simulink model "TrajectoryTracking_2015b_00"  (R2017a)
settings: Solver=ode45  StartTime=0.0  StopTime=200  RelTol=1e-3
values from neighbouring files (symbols this model uses):
  tau_d_1 = C_RB1+C_A1+D1+G1    [DesiredInputOptimalConfiguration.m]
  tau_d_2 = C_RB2+C_A2+D2+G2    [DesiredInputOptimalConfiguration.m]
  tau_d_3 = C_RB3+C_A3+D3+G3    [DesiredInputOptimalConfiguration.m]
  tau_d_4 = C_RB4+C_A4+D4+G4    [DesiredInputOptimalConfiguration.m]
  tau_d_5 = C_RB5+C_A5+D5+G5    [DesiredInputOptimalConfiguration.m]
  tau_d_6 = C_RB6+C_A6+D6+G6    [DesiredInputOptimalConfiguration.m]
  tau_d_7 = C_RB7+C_A7+D7+G7    [DesiredInputOptimalConfiguration.m]
undefined symbols (not defined in the file or in its folder): angular_velocity_pitch_1, angular_velocity_pitch_2, angular_velocity_pitch_3, angular_velocity_pitch_4, angular_velocity_pitch_5, angular_velocity_pitch_6, angular_velocity_roll_1, angular_velocity_roll_2, angular_velocity_roll_3, angular_velocity_roll_4, angular_velocity_roll_5, angular_velocity_roll_6, angular_velocity_roll_7, angular_velocity_yaw_1, angular_velocity_yaw_2, angular_velocity_yaw_3, angular_velocity_yaw_4, angular_velocity_yaw_5, angular_velocity_yaw_6, angular_velocity_yaw_7, B_input, d_H, K1, K2, K3, K4, K5, K6, K7, linear_velocity_x_1, linear_velocity_x_2, linear_velocity_x_3, linear_velocity_x_4, linear_velocity_x_5, linear_velocity_x_6, linear_velocity_x_7, linear_velocity_y_1, linear_velocity_y_2, linear_velocity_y_3, linear_velocity_y_4, linear_velocity_y_5, linear_velocity_y_6, linear_velocity_y_7, linear_velocity_z_1, linear_velocity_z_2, linear_velocity_z_3, linear_velocity_z_4, linear_velocity_z_5, linear_velocity_z_6, linear_velocity_z_7, pitch_angle_1, pitch_angle_2, pitch_angle_3, pitch_angle_4, pitch_angle_5, pitch_angle_6, pitch_angle_7, roll_angle_1, roll_angle_2, roll_angle_3 ... (+54)
undefined symbols (not defined in the file): a_F2, a_F3, a_F4, b_F2, b_F3, b_F4, b_T1_optimized, b_T2_optimized, b_T3_optimized, b_T4_optimized, b_T5_optimized, b_T6_optimized, d_T1_optimized, d_T2_optimized, d_T3_optimized, d_T4_optimized, d_T5_optimized, d_T6_optimized, gamma_F1_optimized, gamma_F2_optimized, gamma_F3_optimized, gamma_F4_optimized, r_T1_optimized, r_T2_optimized, r_T3_optimized, r_T4_optimized, r_T5_optimized, r_T6_optimized, x_F1_optimized, x_F2_optimized, x_F3_optimized, x_F4_optimized
libraries: sharedtransform x1, shared6dofsys x1
(part 2 of 3)

== system TrajectoryTracking_2015b_00/Nonlinear Transformation/Velocity Error /sway_error ==
  sway : Inport
  SwitchSchedule : Inport  Port=2
  Scope3 : Scope  NumInputPorts=2
  Sum5 : Sum  Inputs=|+-
  sway_d : Subsystem
  sway_err : Outport
  wires:
  sway/1 -> Sum5/1
  Sum5/1 -> Scope3/1, sway_err/1
  SwitchSchedule/1 -> sway_d/1(SwitchSchedule)
  sway_d/1(sway_d) -> Scope3/2, Sum5/2

== system TrajectoryTracking_2015b_00/Nonlinear Transformation/Velocity Error /yaw_error ==
  pitch : Inport
  SwitchSchedule : Inport  Port=2
  Scope1 : Scope  NumInputPorts=2
  Scope3 : Scope  NumInputPorts=2
  Sum5 : Sum  Inputs=|+-
  yaw_d : Subsystem
  pitch_err : Outport
  wires:
  pitch/1 -> Scope1/1, Scope3/1, Sum5/1
  Sum5/1 -> pitch_err/1
  yaw_d/1(yaw_d) -> Sum5/2, Scope1/2, Scope3/2
  SwitchSchedule/1 -> yaw_d/1(SwitchSchedule)

== system TrajectoryTracking_2015b_00/Underwater Robot System/Underwater Robot System/DragCalculation ==
  nu : Inport
  Abs : Abs
  Constant : Constant  Value=veh.D
  Product : Product  Multiplication=Matrix(*)
  Product1 : Product
  HullDrag : Outport
  wires:
  Product/1 -> HullDrag/1
  Product1/1 -> Product/2
  Abs/1 -> Product1/1
  Constant/1 -> Product/1
  nu/1 -> Abs/1, Product1/2  "nu"

== system TrajectoryTracking_2015b_00/Underwater Robot System/Underwater Robot System/Dynamic2Kinematic(angular velocity) ==
  "p q r " : Inport
  Initial Integration Phi : Subsystem
  Initial Integration Value Generation Psi : Subsystem
  Initial Integration Value Generation Theta : Subsystem
  Mux1 : Mux  Inputs=3
  Rotation Angles to Direction Cosine Matrix : sharedtransform/Rotation Angles to Direction Cosine Matrix  rotationOrder=ZYX
      settings: SourceProductBaseCode=AE
  Selector : Selector  InputPortWidth=3  IndexOptions=Index vector (dialog)  Indices=[3 2 1]  OutputSizes=1
  phi theta psi : Integrator  InitialConditionSource=external
  phidot thetadot psidot : shared6dofsys/DCM & Euler Angles (Euler)/phidot thetadot psidot
  DCM : Outport
  Euler : Outport  Port=2
  Euler_dot : Outport  Port=3
  wires:
  Selector/1 -> Rotation Angles to Direction Cosine Matrix/1
  "p q r "/1 -> phidot thetadot psidot/1
  phi theta psi/1 -> phidot thetadot psidot/2, Selector/1, Euler/1
  phidot thetadot psidot/1 -> Euler_dot/1, phi theta psi/1
  Rotation Angles to Direction Cosine Matrix/1 -> DCM/1
  Initial Integration Value Generation Psi/1(Initial Orientation Integration Value) -> Mux1/3
  Initial Integration Value Generation Theta/1(Initial Theta Integration Value) -> Mux1/2
  Mux1/1 -> phi theta psi/2
  Initial Integration Phi/1(Initial Phi Integration Value) -> Mux1/1

== system TrajectoryTracking_2015b_00/Underwater Robot System/Underwater Robot System/Initial Integration Value Generation Generalised Location ==
  Constant : Constant  Value=0
  Mux : Mux  Inputs=3
  Initial Location Integration Value : Outport
  wires:
  Constant/1 -> Mux/1, Mux/3, Mux/2
  Mux/1 -> Initial Location Integration Value/1

== system TrajectoryTracking_2015b_00/Underwater Robot System/Underwater Robot System/Underwater Robot Dynamics  ==
  tau_b : Inport
  6DOF Coriolis forces : Subsystem
  M_A : Constant  Value=veh.Ma
  M_RB : Constant  Value=veh.Mrb
  Product : Product  Inputs=/*  Multiplication=Matrix(*)  SaturateOnIntegerOverflow=on  OutDataTypeStr=Inherit: Same as first input
  Scope : Scope
  Selector1 : Selector  InputPortWidth=6  IndexOptions=Index vector (dialog)  Indices=[1 2 3]  OutputSizes=1
  Selector2 : Selector  InputPortWidth=6  IndexOptions=Index vector (dialog)  Indices=[4 5 6]  OutputSizes=1
  Sum : Sum  Inputs=|+-
  Sum2 : Sum  SaturateOnIntegerOverflow=on
  Velocity Integrator : Integrator
  v : Outport
  w_ib : Outport  Port=2
  wires:
  M_RB/1 -> Sum2/1
  M_A/1 -> Sum2/2
  Sum2/1 -> Product/1, 6DOF Coriolis forces/1(M)  "M"
  Selector2/1 -> w_ib/1  "w_nb"
  Product/1 -> Velocity Integrator/1  "(d/dt)nu"
  6DOF Coriolis forces/1(C(nu)nu) -> Sum/2, Scope/1
  Sum/1 -> Product/2
  Selector1/1 -> v/1  "v"
  Velocity Integrator/1 -> 6DOF Coriolis forces/2(nu), Selector2/1, Selector1/1  "nu"
  tau_b/1 -> Sum/1

== system TrajectoryTracking_2015b_00/Underwater Robot System/Underwater Robot System/transform to inertial world frame {i} ==
  v : Inport
  linear velocity transformation matrix : Inport  Port=2
  Product : Product  Multiplication=Matrix(*)  SaturateOnIntegerOverflow=on  InputSameDT=on  OutDataTypeStr=Inherit: Same as first input
  Reshape1 : Reshape  OutputDimensionality=Column vector (2-D)
  Reshape2 : Reshape
  Ve : Outport
  wires:
  Product/1 -> Reshape2/1
  Reshape1/1 -> Product/2
  v/1 -> Reshape1/1
  Reshape2/1 -> Ve/1
  linear velocity transformation matrix/1 -> Product/1

== system TrajectoryTracking_2015b_00/Actuator1/Simplified Fin Model 1/Drag Forces and Moments/3x3 cross product ==
  a : Inport
  b : Inport  Port=2
  Product : Product  SaturateOnIntegerOverflow=on  InputSameDT=on  OutDataTypeStr=Inherit: Same as first input
  Product1 : Product  SaturateOnIntegerOverflow=on  InputSameDT=on  OutDataTypeStr=Inherit: Same as first input
  Selector : Selector  InputPortWidth=3  IndexOptions=Index vector (dialog)  Indices=[2 3 1]  OutputSizes=1
  Selector1 : Selector  InputPortWidth=3  IndexOptions=Index vector (dialog)  Indices=[3 1 2]  OutputSizes=1
  Selector2 : Selector  InputPortWidth=3  IndexOptions=Index vector (dialog)  Indices=[2 3 1]  OutputSizes=1
  Selector3 : Selector  InputPortWidth=3  IndexOptions=Index vector (dialog)  Indices=[3 1 2]  OutputSizes=1
  Sum : Sum  Inputs=+|-  SaturateOnIntegerOverflow=on  InputSameDT=on  OutDataTypeStr=Inherit: Same as first input
  c : Outport  InitialOutput=0
  wires:
  Selector3/1 -> Product1/1
  Selector2/1 -> Product1/2
  Product1/1 -> Sum/2
  Selector1/1 -> Product/2
  Product/1 -> Sum/1
  a/1 -> Selector3/1, Selector/1
  Selector/1 -> Product/1
  b/1 -> Selector2/1, Selector1/1
  Sum/1 -> c/1

== system TrajectoryTracking_2015b_00/Actuator1/Simplified Fin Model 1/Drag Forces and Moments/Drag Force  ==
  AoA : Inport
  u : Inport  Port=2
  Constant : Constant  Value=0
  Gain1 : Gain  Gain=C_D*a_F*b_F
  Mux : Mux  Inputs=3
  Product : Product  Inputs=3
  q(V_ind) : Subsystem
  Drag Force : Outport
  wires:
  Mux/1 -> Drag Force/1
  Gain1/1 -> Product/1
  q(V_ind)/1(q(V_ind)) -> Gain1/1
  Product/1 -> Mux/1
  u/1 -> q(V_ind)/1(u)
  Constant/1 -> Mux/2, Mux/3
  AoA/1 -> Product/3, Product/2

== system TrajectoryTracking_2015b_00/Actuator1/Simplified Fin Model 1/Drag Forces and Moments/Geometric Center of fin ==
  Constant : Constant  Value=gama_F
  Gain : Gain  Gain=0.5*(d_H+a_F)
  Gain1 : Gain  Gain=0.5*(d_H+a_F)
  Mux : Mux  Inputs=3
  Trigonometric Function : Trigonometry  Operator=cos
  Trigonometric Function1 : Trigonometry
  x_F : Constant  Value=x_F
  r_F : Outport
  wires:
  x_F/1 -> Mux/1
  Constant/1 -> Trigonometric Function/1, Trigonometric Function1/1
  Mux/1 -> r_F/1
  Gain/1 -> Mux/2
  Trigonometric Function1/1 -> Gain/1
  Trigonometric Function/1 -> Gain1/1
  Gain1/1 -> Mux/3

== system TrajectoryTracking_2015b_00/Actuator1/Simplified Fin Model 1/Lift Forces and Moments/3x3 cross product ==
  a : Inport
  b : Inport  Port=2
  Product : Product  SaturateOnIntegerOverflow=on  InputSameDT=on  OutDataTypeStr=Inherit: Same as first input
  Product1 : Product  SaturateOnIntegerOverflow=on  InputSameDT=on  OutDataTypeStr=Inherit: Same as first input
  Selector : Selector  InputPortWidth=3  IndexOptions=Index vector (dialog)  Indices=[2 3 1]  OutputSizes=1
  Selector1 : Selector  InputPortWidth=3  IndexOptions=Index vector (dialog)  Indices=[3 1 2]  OutputSizes=1
  Selector2 : Selector  InputPortWidth=3  IndexOptions=Index vector (dialog)  Indices=[2 3 1]  OutputSizes=1
  Selector3 : Selector  InputPortWidth=3  IndexOptions=Index vector (dialog)  Indices=[3 1 2]  OutputSizes=1
  Sum : Sum  Inputs=+|-  SaturateOnIntegerOverflow=on  InputSameDT=on  OutDataTypeStr=Inherit: Same as first input
  c : Outport  InitialOutput=0
  wires:
  Selector3/1 -> Product1/1
  Selector2/1 -> Product1/2
  Product1/1 -> Sum/2
  Selector1/1 -> Product/2
  Product/1 -> Sum/1
  a/1 -> Selector3/1, Selector/1
  Selector/1 -> Product/1
  b/1 -> Selector2/1, Selector1/1
  Sum/1 -> c/1

== system TrajectoryTracking_2015b_00/Actuator1/Simplified Fin Model 1/Lift Forces and Moments/Geometric Center of fin ==
  Constant : Constant  Value=gama_F
  Gain : Gain  Gain=0.5*(d_H+a_F)
  Gain1 : Gain  Gain=0.5*(d_H+a_F)
  Mux : Mux  Inputs=3
  Trigonometric Function : Trigonometry  Operator=cos
  Trigonometric Function1 : Trigonometry
  x_F : Constant  Value=x_F
  r_F : Outport
  wires:
  x_F/1 -> Mux/1
  Constant/1 -> Trigonometric Function/1, Trigonometric Function1/1
  Mux/1 -> r_F/1
  Gain/1 -> Mux/2
  Trigonometric Function1/1 -> Gain/1
  Trigonometric Function/1 -> Gain1/1
  Gain1/1 -> Mux/3

== system TrajectoryTracking_2015b_00/Actuator1/Simplified Fin Model 1/Lift Forces and Moments/Lift Force  ==
  u : Inport
  AoA : Inport  Port=2
  Constant : Constant  Value=0
  Constant1 : Constant  Value=gama_F
  Gain1 : Gain  Gain=C_L*a_F*b_F
  Gain2 : Gain  Gain=-C_L*a_F*b_F
  Mux : Mux  Inputs=3
  Product : Product  Inputs=3
  Product1 : Product  Inputs=3
  Trigonometric Function : Trigonometry  Operator=cos
  Trigonometric Function1 : Trigonometry
  q(V_ind) : Subsystem
  Lift Force : Outport
  wires:
  u/1 -> q(V_ind)/1(u)
  q(V_ind)/1(q(V_ind)) -> Gain2/1, Gain1/1
  Gain1/1 -> Product/1
  Trigonometric Function/1 -> Product/2
  Mux/1 -> Lift Force/1
  Gain2/1 -> Product1/1
  Trigonometric Function1/1 -> Product1/2
  Constant/1 -> Mux/1
  Product/1 -> Mux/2
  Product1/1 -> Mux/3
  AoA/1 -> Product/3, Product1/3
  Constant1/1 -> Trigonometric Function1/1, Trigonometric Function/1

== system TrajectoryTracking_2015b_00/Actuator1/Simplified Fin Model 2/Drag Forces and Moments/3x3 cross product ==
  a : Inport
  b : Inport  Port=2
  Product : Product  SaturateOnIntegerOverflow=on  InputSameDT=on  OutDataTypeStr=Inherit: Same as first input
  Product1 : Product  SaturateOnIntegerOverflow=on  InputSameDT=on  OutDataTypeStr=Inherit: Same as first input
  Selector : Selector  InputPortWidth=3  IndexOptions=Index vector (dialog)  Indices=[2 3 1]  OutputSizes=1
  Selector1 : Selector  InputPortWidth=3  IndexOptions=Index vector (dialog)  Indices=[3 1 2]  OutputSizes=1
  Selector2 : Selector  InputPortWidth=3  IndexOptions=Index vector (dialog)  Indices=[2 3 1]  OutputSizes=1
  Selector3 : Selector  InputPortWidth=3  IndexOptions=Index vector (dialog)  Indices=[3 1 2]  OutputSizes=1
  Sum : Sum  Inputs=+|-  SaturateOnIntegerOverflow=on  InputSameDT=on  OutDataTypeStr=Inherit: Same as first input
  c : Outport  InitialOutput=0
  wires:
  Selector3/1 -> Product1/1
  Selector2/1 -> Product1/2
  Product1/1 -> Sum/2
  Selector1/1 -> Product/2
  Product/1 -> Sum/1
  a/1 -> Selector3/1, Selector/1
  Selector/1 -> Product/1
  b/1 -> Selector2/1, Selector1/1
  Sum/1 -> c/1

== system TrajectoryTracking_2015b_00/Actuator1/Simplified Fin Model 2/Drag Forces and Moments/Drag Force  ==
  AoA : Inport
  u : Inport  Port=2
  Constant : Constant  Value=0
  Gain1 : Gain  Gain=C_D*a_F*b_F
  Mux : Mux  Inputs=3
  Product : Product  Inputs=3
  q(V_ind) : Subsystem
  Drag Force : Outport
  wires:
  Mux/1 -> Drag Force/1
  Gain1/1 -> Product/1
  q(V_ind)/1(q(V_ind)) -> Gain1/1
  Product/1 -> Mux/1
  u/1 -> q(V_ind)/1(u)
  Constant/1 -> Mux/2, Mux/3
  AoA/1 -> Product/3, Product/2

== system TrajectoryTracking_2015b_00/Actuator1/Simplified Fin Model 2/Drag Forces and Moments/Geometric Center of fin ==
  Constant : Constant  Value=gama_F
  Gain : Gain  Gain=0.5*(d_H+a_F)
  Gain1 : Gain  Gain=0.5*(d_H+a_F)
  Mux : Mux  Inputs=3
  Trigonometric Function : Trigonometry  Operator=cos
  Trigonometric Function1 : Trigonometry
  x_F : Constant  Value=x_F
  r_F : Outport
  wires:
  x_F/1 -> Mux/1
  Constant/1 -> Trigonometric Function/1, Trigonometric Function1/1
  Mux/1 -> r_F/1
  Gain/1 -> Mux/2
  Trigonometric Function1/1 -> Gain/1
  Trigonometric Function/1 -> Gain1/1
  Gain1/1 -> Mux/3

== system TrajectoryTracking_2015b_00/Actuator1/Simplified Fin Model 2/Lift Forces and Moments/3x3 cross product ==
  a : Inport
  b : Inport  Port=2
  Product : Product  SaturateOnIntegerOverflow=on  InputSameDT=on  OutDataTypeStr=Inherit: Same as first input
  Product1 : Product  SaturateOnIntegerOverflow=on  InputSameDT=on  OutDataTypeStr=Inherit: Same as first input
  Selector : Selector  InputPortWidth=3  IndexOptions=Index vector (dialog)  Indices=[2 3 1]  OutputSizes=1
  Selector1 : Selector  InputPortWidth=3  IndexOptions=Index vector (dialog)  Indices=[3 1 2]  OutputSizes=1
  Selector2 : Selector  InputPortWidth=3  IndexOptions=Index vector (dialog)  Indices=[2 3 1]  OutputSizes=1
  Selector3 : Selector  InputPortWidth=3  IndexOptions=Index vector (dialog)  Indices=[3 1 2]  OutputSizes=1
  Sum : Sum  Inputs=+|-  SaturateOnIntegerOverflow=on  InputSameDT=on  OutDataTypeStr=Inherit: Same as first input
  c : Outport  InitialOutput=0
  wires:
  Selector3/1 -> Product1/1
  Selector2/1 -> Product1/2
  Product1/1 -> Sum/2
  Selector1/1 -> Product/2
  Product/1 -> Sum/1
  a/1 -> Selector3/1, Selector/1
  Selector/1 -> Product/1
  b/1 -> Selector2/1, Selector1/1
  Sum/1 -> c/1

== system TrajectoryTracking_2015b_00/Actuator1/Simplified Fin Model 2/Lift Forces and Moments/Geometric Center of fin ==
  Constant : Constant  Value=gama_F
  Gain : Gain  Gain=0.5*(d_H+a_F)
  Gain1 : Gain  Gain=0.5*(d_H+a_F)
  Mux : Mux  Inputs=3
  Trigonometric Function : Trigonometry  Operator=cos
  Trigonometric Function1 : Trigonometry
  x_F : Constant  Value=x_F
  r_F : Outport
  wires:
  x_F/1 -> Mux/1
  Constant/1 -> Trigonometric Function/1, Trigonometric Function1/1
  Mux/1 -> r_F/1
  Gain/1 -> Mux/2
  Trigonometric Function1/1 -> Gain/1
  Trigonometric Function/1 -> Gain1/1
  Gain1/1 -> Mux/3

== system TrajectoryTracking_2015b_00/Actuator1/Simplified Fin Model 2/Lift Forces and Moments/Lift Force  ==
  u : Inport
  AoA : Inport  Port=2
  Constant : Constant  Value=0
  Constant1 : Constant  Value=gama_F
  Gain1 : Gain  Gain=C_L*a_F*b_F
  Gain2 : Gain  Gain=-C_L*a_F*b_F
  Mux : Mux  Inputs=3
  Product : Product  Inputs=3
  Product1 : Product  Inputs=3
  Trigonometric Function : Trigonometry  Operator=cos
  Trigonometric Function1 : Trigonometry
  q(V_ind) : Subsystem
  Lift Force : Outport
  wires:
  u/1 -> q(V_ind)/1(u)
  q(V_ind)/1(q(V_ind)) -> Gain2/1, Gain1/1
  Gain1/1 -> Product/1
  Trigonometric Function/1 -> Product/2
  Mux/1 -> Lift Force/1
  Gain2/1 -> Product1/1
  Trigonometric Function1/1 -> Product1/2
  Constant/1 -> Mux/1
  Product/1 -> Mux/2
  Product1/1 -> Mux/3
  AoA/1 -> Product/3, Product1/3
  Constant1/1 -> Trigonometric Function1/1, Trigonometric Function/1

== system TrajectoryTracking_2015b_00/Actuator1/Simplified Fin Model 3/Drag Forces and Moments/3x3 cross product ==
  a : Inport
  b : Inport  Port=2
  Product : Product  SaturateOnIntegerOverflow=on  InputSameDT=on  OutDataTypeStr=Inherit: Same as first input
  Product1 : Product  SaturateOnIntegerOverflow=on  InputSameDT=on  OutDataTypeStr=Inherit: Same as first input
  Selector : Selector  InputPortWidth=3  IndexOptions=Index vector (dialog)  Indices=[2 3 1]  OutputSizes=1
  Selector1 : Selector  InputPortWidth=3  IndexOptions=Index vector (dialog)  Indices=[3 1 2]  OutputSizes=1
  Selector2 : Selector  InputPortWidth=3  IndexOptions=Index vector (dialog)  Indices=[2 3 1]  OutputSizes=1
  Selector3 : Selector  InputPortWidth=3  IndexOptions=Index vector (dialog)  Indices=[3 1 2]  OutputSizes=1
  Sum : Sum  Inputs=+|-  SaturateOnIntegerOverflow=on  InputSameDT=on  OutDataTypeStr=Inherit: Same as first input
  c : Outport  InitialOutput=0
  wires:
  Selector3/1 -> Product1/1
  Selector2/1 -> Product1/2
  Product1/1 -> Sum/2
  Selector1/1 -> Product/2
  Product/1 -> Sum/1
  a/1 -> Selector3/1, Selector/1
  Selector/1 -> Product/1
  b/1 -> Selector2/1, Selector1/1
  Sum/1 -> c/1

== system TrajectoryTracking_2015b_00/Actuator1/Simplified Fin Model 3/Drag Forces and Moments/Drag Force  ==
  AoA : Inport
  u : Inport  Port=2
  Constant : Constant  Value=0
  Gain1 : Gain  Gain=C_D*a_F*b_F
  Mux : Mux  Inputs=3
  Product : Product  Inputs=3
  q(V_ind) : Subsystem
  Drag Force : Outport
  wires:
  Mux/1 -> Drag Force/1
  Gain1/1 -> Product/1
  q(V_ind)/1(q(V_ind)) -> Gain1/1
  Product/1 -> Mux/1
  u/1 -> q(V_ind)/1(u)
  Constant/1 -> Mux/2, Mux/3
  AoA/1 -> Product/3, Product/2

== system TrajectoryTracking_2015b_00/Actuator1/Simplified Fin Model 3/Drag Forces and Moments/Geometric Center of fin ==
  Constant : Constant  Value=gama_F
  Gain : Gain  Gain=0.5*(d_H+a_F)
  Gain1 : Gain  Gain=0.5*(d_H+a_F)
  Mux : Mux  Inputs=3
  Trigonometric Function : Trigonometry  Operator=cos
  Trigonometric Function1 : Trigonometry
  x_F : Constant  Value=x_F
  r_F : Outport
  wires:
  x_F/1 -> Mux/1
  Constant/1 -> Trigonometric Function/1, Trigonometric Function1/1
  Mux/1 -> r_F/1
  Gain/1 -> Mux/2
  Trigonometric Function1/1 -> Gain/1
  Trigonometric Function/1 -> Gain1/1
  Gain1/1 -> Mux/3

== system TrajectoryTracking_2015b_00/Actuator1/Simplified Fin Model 3/Lift Forces and Moments/3x3 cross product ==
  a : Inport
  b : Inport  Port=2
  Product : Product  SaturateOnIntegerOverflow=on  InputSameDT=on  OutDataTypeStr=Inherit: Same as first input
  Product1 : Product  SaturateOnIntegerOverflow=on  InputSameDT=on  OutDataTypeStr=Inherit: Same as first input
  Selector : Selector  InputPortWidth=3  IndexOptions=Index vector (dialog)  Indices=[2 3 1]  OutputSizes=1
  Selector1 : Selector  InputPortWidth=3  IndexOptions=Index vector (dialog)  Indices=[3 1 2]  OutputSizes=1
  Selector2 : Selector  InputPortWidth=3  IndexOptions=Index vector (dialog)  Indices=[2 3 1]  OutputSizes=1
  Selector3 : Selector  InputPortWidth=3  IndexOptions=Index vector (dialog)  Indices=[3 1 2]  OutputSizes=1
  Sum : Sum  Inputs=+|-  SaturateOnIntegerOverflow=on  InputSameDT=on  OutDataTypeStr=Inherit: Same as first input
  c : Outport  InitialOutput=0
  wires:
  Selector3/1 -> Product1/1
  Selector2/1 -> Product1/2
  Product1/1 -> Sum/2
  Selector1/1 -> Product/2
  Product/1 -> Sum/1
  a/1 -> Selector3/1, Selector/1
  Selector/1 -> Product/1
  b/1 -> Selector2/1, Selector1/1
  Sum/1 -> c/1

== system TrajectoryTracking_2015b_00/Actuator1/Simplified Fin Model 3/Lift Forces and Moments/Geometric Center of fin ==
  Constant : Constant  Value=gama_F
  Gain : Gain  Gain=0.5*(d_H+a_F)
  Gain1 : Gain  Gain=0.5*(d_H+a_F)
  Mux : Mux  Inputs=3
  Trigonometric Function : Trigonometry  Operator=cos
  Trigonometric Function1 : Trigonometry
  x_F : Constant  Value=x_F
  r_F : Outport
  wires:
  x_F/1 -> Mux/1
  Constant/1 -> Trigonometric Function/1, Trigonometric Function1/1
  Mux/1 -> r_F/1
  Gain/1 -> Mux/2
  Trigonometric Function1/1 -> Gain/1
  Trigonometric Function/1 -> Gain1/1
  Gain1/1 -> Mux/3

== system TrajectoryTracking_2015b_00/Actuator1/Simplified Fin Model 3/Lift Forces and Moments/Lift Force  ==
  u : Inport
  AoA : Inport  Port=2
  Constant : Constant  Value=0
  Constant1 : Constant  Value=gama_F
  Gain1 : Gain  Gain=C_L*a_F*b_F
  Gain2 : Gain  Gain=-C_L*a_F*b_F
  Mux : Mux  Inputs=3
  Product : Product  Inputs=3
  Product1 : Product  Inputs=3
  Trigonometric Function : Trigonometry  Operator=cos
  Trigonometric Function1 : Trigonometry
  q(V_ind) : Subsystem
  Lift Force : Outport
  wires:
  u/1 -> q(V_ind)/1(u)
  q(V_ind)/1(q(V_ind)) -> Gain2/1, Gain1/1
  Gain1/1 -> Product/1
  Trigonometric Function/1 -> Product/2
  Mux/1 -> Lift Force/1
  Gain2/1 -> Product1/1
  Trigonometric Function1/1 -> Product1/2
  Constant/1 -> Mux/1
  Product/1 -> Mux/2
  Product1/1 -> Mux/3
  AoA/1 -> Product/3, Product1/3
  Constant1/1 -> Trigonometric Function1/1, Trigonometric Function/1

== system TrajectoryTracking_2015b_00/Actuator1/Simplified Fin Model 4/Drag Forces and Moments/3x3 cross product ==
  a : Inport
  b : Inport  Port=2
  Product : Product  SaturateOnIntegerOverflow=on  InputSameDT=on  OutDataTypeStr=Inherit: Same as first input
  Product1 : Product  SaturateOnIntegerOverflow=on  InputSameDT=on  OutDataTypeStr=Inherit: Same as first input
  Selector : Selector  InputPortWidth=3  IndexOptions=Index vector (dialog)  Indices=[2 3 1]  OutputSizes=1
  Selector1 : Selector  InputPortWidth=3  IndexOptions=Index vector (dialog)  Indices=[3 1 2]  OutputSizes=1
  Selector2 : Selector  InputPortWidth=3  IndexOptions=Index vector (dialog)  Indices=[2 3 1]  OutputSizes=1
  Selector3 : Selector  InputPortWidth=3  IndexOptions=Index vector (dialog)  Indices=[3 1 2]  OutputSizes=1
  Sum : Sum  Inputs=+|-  SaturateOnIntegerOverflow=on  InputSameDT=on  OutDataTypeStr=Inherit: Same as first input
  c : Outport  InitialOutput=0
  wires:
  Selector3/1 -> Product1/1
  Selector2/1 -> Product1/2
  Product1/1 -> Sum/2
  Selector1/1 -> Product/2
  Product/1 -> Sum/1
  a/1 -> Selector3/1, Selector/1
  Selector/1 -> Product/1
  b/1 -> Selector2/1, Selector1/1
  Sum/1 -> c/1

== system TrajectoryTracking_2015b_00/Actuator1/Simplified Fin Model 4/Drag Forces and Moments/Drag Force  ==
  AoA : Inport
  u : Inport  Port=2
  Constant : Constant  Value=0
  Gain1 : Gain  Gain=C_D*a_F*b_F
  Mux : Mux  Inputs=3
  Product : Product  Inputs=3
  q(V_ind) : Subsystem
  Drag Force : Outport
  wires:
  Mux/1 -> Drag Force/1
  Gain1/1 -> Product/1
  q(V_ind)/1(q(V_ind)) -> Gain1/1
  Product/1 -> Mux/1
  u/1 -> q(V_ind)/1(u)
  Constant/1 -> Mux/2, Mux/3
  AoA/1 -> Product/3, Product/2

== system TrajectoryTracking_2015b_00/Actuator1/Simplified Fin Model 4/Drag Forces and Moments/Geometric Center of fin ==
  Constant : Constant  Value=gama_F
  Gain : Gain  Gain=0.5*(d_H+a_F)
  Gain1 : Gain  Gain=0.5*(d_H+a_F)
  Mux : Mux  Inputs=3
  Trigonometric Function : Trigonometry  Operator=cos
  Trigonometric Function1 : Trigonometry
  x_F : Constant  Value=x_F
  r_F : Outport
  wires:
  x_F/1 -> Mux/1
  Constant/1 -> Trigonometric Function/1, Trigonometric Function1/1
  Mux/1 -> r_F/1
  Gain/1 -> Mux/2
  Trigonometric Function1/1 -> Gain/1
  Trigonometric Function/1 -> Gain1/1
  Gain1/1 -> Mux/3

== system TrajectoryTracking_2015b_00/Actuator1/Simplified Fin Model 4/Lift Forces and Moments/3x3 cross product ==
  a : Inport
  b : Inport  Port=2
  Product : Product  SaturateOnIntegerOverflow=on  InputSameDT=on  OutDataTypeStr=Inherit: Same as first input
  Product1 : Product  SaturateOnIntegerOverflow=on  InputSameDT=on  OutDataTypeStr=Inherit: Same as first input
  Selector : Selector  InputPortWidth=3  IndexOptions=Index vector (dialog)  Indices=[2 3 1]  OutputSizes=1
  Selector1 : Selector  InputPortWidth=3  IndexOptions=Index vector (dialog)  Indices=[3 1 2]  OutputSizes=1
  Selector2 : Selector  InputPortWidth=3  IndexOptions=Index vector (dialog)  Indices=[2 3 1]  OutputSizes=1
  Selector3 : Selector  InputPortWidth=3  IndexOptions=Index vector (dialog)  Indices=[3 1 2]  OutputSizes=1
  Sum : Sum  Inputs=+|-  SaturateOnIntegerOverflow=on  InputSameDT=on  OutDataTypeStr=Inherit: Same as first input
  c : Outport  InitialOutput=0
  wires:
  Selector3/1 -> Product1/1
  Selector2/1 -> Product1/2
  Product1/1 -> Sum/2
  Selector1/1 -> Product/2
  Product/1 -> Sum/1
  a/1 -> Selector3/1, Selector/1
  Selector/1 -> Product/1
  b/1 -> Selector2/1, Selector1/1
  Sum/1 -> c/1

== system TrajectoryTracking_2015b_00/Actuator1/Simplified Fin Model 4/Lift Forces and Moments/Geometric Center of fin ==
  Constant : Constant  Value=gama_F
  Gain : Gain  Gain=0.5*(d_H+a_F)
  Gain1 : Gain  Gain=0.5*(d_H+a_F)
  Mux : Mux  Inputs=3
  Trigonometric Function : Trigonometry  Operator=cos
  Trigonometric Function1 : Trigonometry
  x_F : Constant  Value=x_F
  r_F : Outport
  wires:
  x_F/1 -> Mux/1
  Constant/1 -> Trigonometric Function/1, Trigonometric Function1/1
  Mux/1 -> r_F/1
  Gain/1 -> Mux/2
  Trigonometric Function1/1 -> Gain/1
  Trigonometric Function/1 -> Gain1/1
  Gain1/1 -> Mux/3

== system TrajectoryTracking_2015b_00/Actuator1/Simplified Fin Model 4/Lift Forces and Moments/Lift Force  ==
  u : Inport
  AoA : Inport  Port=2
  Constant : Constant  Value=0
  Constant1 : Constant  Value=gama_F
  Gain1 : Gain  Gain=C_L*a_F*b_F
  Gain2 : Gain  Gain=-C_L*a_F*b_F
  Mux : Mux  Inputs=3
  Product : Product  Inputs=3
  Product1 : Product  Inputs=3
  Trigonometric Function : Trigonometry  Operator=cos
  Trigonometric Function1 : Trigonometry
  q(V_ind) : Subsystem
  Lift Force : Outport
  wires:
  u/1 -> q(V_ind)/1(u)
  q(V_ind)/1(q(V_ind)) -> Gain2/1, Gain1/1
  Gain1/1 -> Product/1
  Trigonometric Function/1 -> Product/2
  Mux/1 -> Lift Force/1
  Gain2/1 -> Product1/1
  Trigonometric Function1/1 -> Product1/2
  Constant/1 -> Mux/1
  Product/1 -> Mux/2
  Product1/1 -> Mux/3
  AoA/1 -> Product/3, Product1/3
  Constant1/1 -> Trigonometric Function1/1, Trigonometric Function/1

== system TrajectoryTracking_2015b_00/Nonlinear Transformation/Position Error /Nonlinear Orientation Transformation/Euler Angles to Angular Velocity Transfomration matrix ==
  theta : Inport
  Constant : Constant
  Constant1 : Constant  Value=0
  Mux : Mux  Inputs=9
  Reshape : Reshape  OutputDimensionality=Customize  OutputDimensions=[3,3]
  T21 : Fcn  Expr=sin(u(1))*tan(u(2))
  T22 : Fcn  Expr=cos(u(1))
  T23 : Fcn  Expr=sin(u(1))/cos(u(2))
  T31 : Fcn  Expr=cos(u(1))*tan(u(2))
  T32 : Fcn  Expr=-sin(u(1))
  T33 : Fcn  Expr=cos(u(1))/cos(u(2))
  T : Outport
  wires:
  Mux/1 -> Reshape/1
  Constant/1 -> Mux/1
  Constant1/1 -> Mux/2, Mux/3
  T21/1 -> Mux/4
  theta/1 -> T23/1, T33/1, T32/1, T31/1, T21/1, T22/1
  T22/1 -> Mux/5
  T23/1 -> Mux/6
  T31/1 -> Mux/7
  T32/1 -> Mux/8
  T33/1 -> Mux/9
  Reshape/1 -> T/1

== system TrajectoryTracking_2015b_00/Nonlinear Transformation/Position Error /Nonlinear Orientation Transformation/pitch_error ==
  pitch : Inport
  SwitchSchedule : Inport  Port=2
  Scope2 : Scope  NumInputPorts=2
  Sum13 : Sum  Inputs=|+-
  To Workspace : ToWorkspace  VariableName=theta_s  SaveFormat=Timeseries  SampleTime=-1
  theta_d : Subsystem
  pitch_err : Outport
  wires:
  pitch/1 -> To Workspace/1, Scope2/1, Sum13/1
  Sum13/1 -> pitch_err/1
  SwitchSchedule/1 -> theta_d/1(SwitchSchedule)
  theta_d/1(theta_d) -> Sum13/2, Scope2/2

== system TrajectoryTracking_2015b_00/Nonlinear Transformation/Position Error /Nonlinear Orientation Transformation/roll_error ==
  roll : Inport
  SwitchSchedule : Inport  Port=2
  Scope2 : Scope  NumInputPorts=2
  Sum13 : Sum  Inputs=|+-
  To Workspace : ToWorkspace  VariableName=phi_s  SaveFormat=Timeseries  SampleTime=-1
  phi_d : Subsystem
  roll_err : Outport
  wires:
  roll/1 -> To Workspace/1, Scope2/1, Sum13/1
  Sum13/1 -> roll_err/1
  SwitchSchedule/1 -> phi_d/1(SwitchSchedule)
  phi_d/1(phi_d) -> Scope2/2, Sum13/2

== system TrajectoryTracking_2015b_00/Nonlinear Transformation/Position Error /Nonlinear Orientation Transformation/yaw_error ==
  yaw : Inport
  SwitchSchedule : Inport  Port=2
  Scope2 : Scope  NumInputPorts=2
  Sum13 : Sum  Inputs=|+-
  To Workspace : ToWorkspace  VariableName=psi_s  SaveFormat=Timeseries  SampleTime=-1
  theta_d : Subsystem
  yaw_err : Outport
  wires:
  yaw/1 -> To Workspace/1, Scope2/1, Sum13/1
  Sum13/1 -> yaw_err/1
  theta_d/1(yaw_d) -> Scope2/2, Sum13/2
  SwitchSchedule/1 -> theta_d/1(SwitchSchedule)

== system TrajectoryTracking_2015b_00/Nonlinear Transformation/Position Error /Nonlinear Position Transformation/Euler Angles to inverse rotation matrix ==
  theta : Inport
  Mux : Mux  Inputs=2
  Mux1 : Mux  Inputs=9
  R11 : Fcn  Expr=u(5)*u(6)
  R12 : Fcn  Expr=u(5)*u(3)
  R13 : Fcn  Expr=-u(2)
  R21 : Fcn  Expr=-u(4)*u(3)+u(1)*u(2)*u(6)
  R22 : Fcn  Expr=u(4)*u(6)+u(1)*u(2)*u(3)
  R23 : Fcn  Expr=u(1)*u(5)
  R31 : Fcn  Expr=u(1)*u(3)+u(4)*u(2)*u(6)
  R32 : Fcn  Expr=-u(1)*u(6)+u(4)*u(2)*u(3)
  R33 : Fcn  Expr=u(4)*u(5)
  Reshape : Reshape  OutputDimensionality=Customize  OutputDimensions=[3,3]
  Trigonometric Function1 : Trigonometry  Operator=cos
  sin(theta) : Trigonometry
  inv(R) : Outport
  wires:
  theta/1 -> Trigonometric Function1/1, sin(theta)/1
  Trigonometric Function1/1 -> Mux/2
  sin(theta)/1 -> Mux/1
  Mux1/1 -> Reshape/1
  Mux/1 -> R32/1, R33/1, R23/1, R13/1, R22/1, R12/1, R31/1, R11/1, R21/1
  R11/1 -> Mux1/1
  R21/1 -> Mux1/2
  R31/1 -> Mux1/3
  R12/1 -> Mux1/4
  R22/1 -> Mux1/5
  R32/1 -> Mux1/6
  R13/1 -> Mux1/7
  R23/1 -> Mux1/8
  R33/1 -> Mux1/9
  Reshape/1 -> inv(R)/1

== system TrajectoryTracking_2015b_00/Nonlinear Transformation/Position Error /Nonlinear Position Transformation/x_error ==
  x : Inport
  SwitchSchedule : Inport  Port=2
  Scope2 : Scope  NumInputPorts=2
  Sum11 : Sum  Inputs=|+-
  To Workspace : ToWorkspace  VariableName=x_s  SaveFormat=Timeseries  SampleTime=-1
  To Workspace1 : ToWorkspace  VariableName=x_r  SaveFormat=Timeseries  SampleTime=-1
  x_d : Subsystem
  x_err : Outport
  wires:
  x/1 -> To Workspace/1, Scope2/1, Sum11/1
  Sum11/1 -> x_err/1
  SwitchSchedule/1 -> x_d/1(SwitchSchedule)
  x_d/1(x_d) -> Sum11/2, To Workspace1/1, Scope2/2

== system TrajectoryTracking_2015b_00/Nonlinear Transformation/Position Error /Nonlinear Position Transformation/y_error ==
  y : Inport
  SwitchSchedule : Inport  Port=2
  Scope2 : Scope  NumInputPorts=2
  Sum12 : Sum  Inputs=|+-
  To Workspace : ToWorkspace  VariableName=y_s  SaveFormat=Timeseries  SampleTime=-1
  To Workspace1 : ToWorkspace  VariableName=y_r  SaveFormat=Timeseries  SampleTime=-1
  y_d : Subsystem
  y_err : Outport
  wires:
  y/1 -> To Workspace/1, Scope2/1, Sum12/1
  Sum12/1 -> y_err/1
  SwitchSchedule/1 -> y_d/1(SwitchSchedule)
  y_d/1(y_d) -> To Workspace1/1, Sum12/2, Scope2/2

== system TrajectoryTracking_2015b_00/Nonlinear Transformation/Position Error /Nonlinear Position Transformation/z_error ==
  z : Inport
  SwitchSchedule : Inport  Port=2
  Scope2 : Scope  NumInputPorts=2
  Sum13 : Sum  Inputs=|+-
  To Workspace : ToWorkspace  VariableName=z_s  SaveFormat=Timeseries  SampleTime=-1
  To Workspace1 : ToWorkspace  VariableName=z_r  SaveFormat=Timeseries  SampleTime=-1
  z_d : Subsystem
  z_err : Outport
  wires:
  z/1 -> To Workspace/1, Scope2/1, Sum13/1
  Sum13/1 -> z_err/1
  SwitchSchedule/1 -> z_d/1(SwitchSchedule)
  z_d/1(z_d) -> To Workspace1/1, Scope2/2, Sum13/2

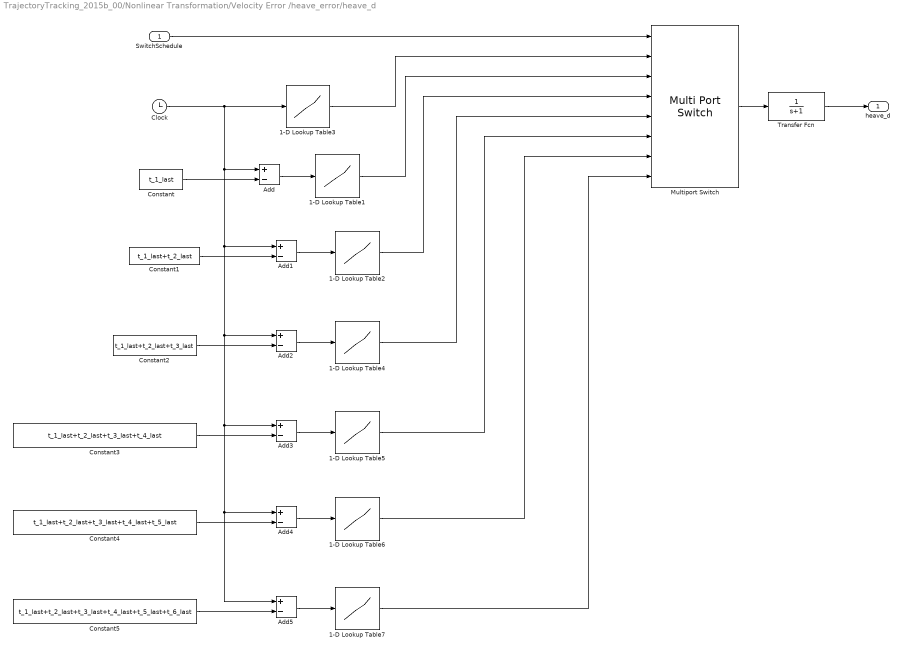
== system TrajectoryTracking_2015b_00/Nonlinear Transformation/Velocity Error /heave_error/heave_d ==
  SwitchSchedule : Inport
  1-D Lookup Table1 : Lookup_n-D  NumberOfTableDimensions=1  BreakpointsForDimension1=t_e_2  Table=linear_velocity_z_2  InternalRulePriority=Speed  RndMeth=Simplest  InputSameDT=on
  1-D Lookup Table2 : Lookup_n-D  NumberOfTableDimensions=1  BreakpointsForDimension1=t_e_3  Table=linear_velocity_z_3  InternalRulePriority=Speed  RndMeth=Simplest  InputSameDT=on
  1-D Lookup Table3 : Lookup_n-D  NumberOfTableDimensions=1  BreakpointsForDimension1=t_e_1  Table=linear_velocity_z_1  InternalRulePriority=Speed  RndMeth=Simplest  InputSameDT=on
  1-D Lookup Table4 : Lookup_n-D  NumberOfTableDimensions=1  BreakpointsForDimension1=t_e_4  Table=linear_velocity_z_4  InternalRulePriority=Speed  RndMeth=Simplest  InputSameDT=on
  1-D Lookup Table5 : Lookup_n-D  NumberOfTableDimensions=1  BreakpointsForDimension1=t_e_5  Table=linear_velocity_z_5  InternalRulePriority=Speed  RndMeth=Simplest  InputSameDT=on
  1-D Lookup Table6 : Lookup_n-D  NumberOfTableDimensions=1  BreakpointsForDimension1=t_e_6  Table=linear_velocity_z_6  InternalRulePriority=Speed  RndMeth=Simplest  InputSameDT=on
  1-D Lookup Table7 : Lookup_n-D  NumberOfTableDimensions=1  BreakpointsForDimension1=t_e_7  Table=linear_velocity_z_7  InternalRulePriority=Speed  RndMeth=Simplest  InputSameDT=on
  Add{,1..5} (6 alike) : Sum  Inputs=+-
  Clock : Clock
  Constant : Constant  Value=t_1_last
  Constant1 : Constant  Value=t_1_last+t_2_last
  Constant2 : Constant  Value=t_1_last+t_2_last+t_3_last
  Constant3 : Constant  Value=t_1_last+t_2_last+t_3_last+t_4_last
  Constant4 : Constant  Value=t_1_last+t_2_last+t_3_last+t_4_last+t_5_last
  Constant5 : Constant  Value=t_1_last+t_2_last+t_3_last+t_4_last+t_5_last+t_6_last
  Multiport Switch : MultiPortSwitch  Inputs=7
  Transfer Fcn : TransferFcn  Denominator=[1 1]
  heave_d : Outport
  wires:
  1-D Lookup Table1/1 -> Multiport Switch/3
  1-D Lookup Table3/1 -> Multiport Switch/2
  Constant/1 -> Add/2
  Multiport Switch/1 -> Transfer Fcn/1
  SwitchSchedule/1 -> Multiport Switch/1
  Add/1 -> 1-D Lookup Table1/1
  Constant1/1 -> Add1/2
  Add1/1 -> 1-D Lookup Table2/1
  1-D Lookup Table2/1 -> Multiport Switch/4
  Clock/1 -> Add5/1, Add4/1, Add3/1, Add2/1, Add1/1, Add/1, 1-D Lookup Table3/1
  Add2/1 -> 1-D Lookup Table4/1
  Constant2/1 -> Add2/2
  1-D Lookup Table4/1 -> Multiport Switch/5
  Transfer Fcn/1 -> heave_d/1
  Add3/1 -> 1-D Lookup Table5/1
  Constant3/1 -> Add3/2
  1-D Lookup Table5/1 -> Multiport Switch/6
  Add4/1 -> 1-D Lookup Table6/1
  Constant4/1 -> Add4/2
  1-D Lookup Table6/1 -> Multiport Switch/7
  Add5/1 -> 1-D Lookup Table7/1
  Constant5/1 -> Add5/2
  1-D Lookup Table7/1 -> Multiport Switch/8

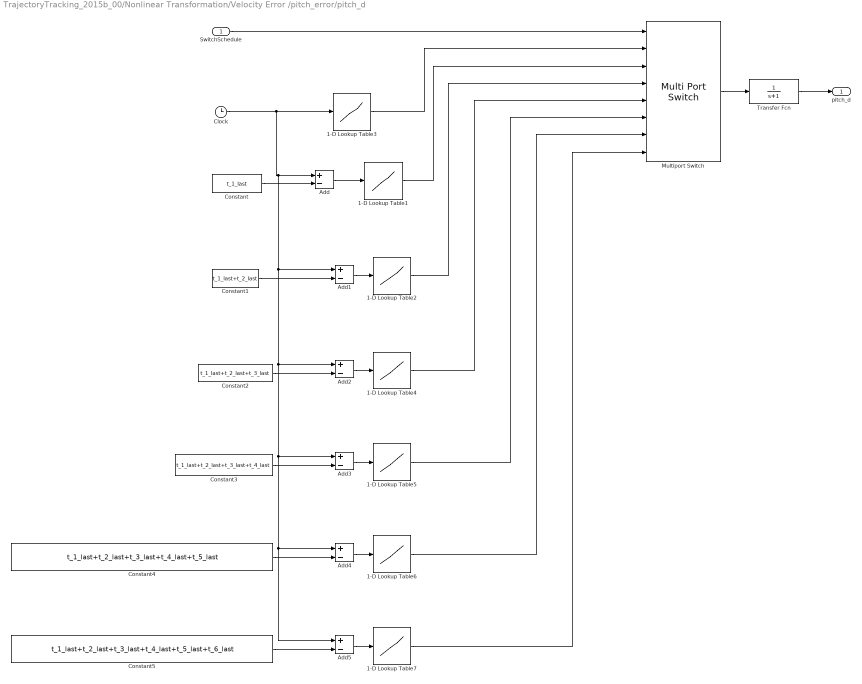
== system TrajectoryTracking_2015b_00/Nonlinear Transformation/Velocity Error /pitch_error/pitch_d ==
  SwitchSchedule : Inport
  1-D Lookup Table1 : Lookup_n-D  NumberOfTableDimensions=1  BreakpointsForDimension1=t_e_2  Table=angular_velocity_pitch_2  InternalRulePriority=Speed  RndMeth=Simplest  InputSameDT=on
  1-D Lookup Table2 : Lookup_n-D  NumberOfTableDimensions=1  BreakpointsForDimension1=t_e_3  Table=angular_velocity_pitch_3  InternalRulePriority=Speed  RndMeth=Simplest  InputSameDT=on
  1-D Lookup Table3 : Lookup_n-D  NumberOfTableDimensions=1  BreakpointsForDimension1=t_e_1  Table=angular_velocity_pitch_1  InternalRulePriority=Speed  RndMeth=Simplest  InputSameDT=on
  1-D Lookup Table4 : Lookup_n-D  NumberOfTableDimensions=1  BreakpointsForDimension1=t_e_4  Table=angular_velocity_pitch_4  InternalRulePriority=Speed  RndMeth=Simplest  InputSameDT=on
  1-D Lookup Table5 : Lookup_n-D  NumberOfTableDimensions=1  BreakpointsForDimension1=t_e_5  Table=angular_velocity_pitch_5  InternalRulePriority=Speed  RndMeth=Simplest  InputSameDT=on
  1-D Lookup Table6 : Lookup_n-D  NumberOfTableDimensions=1  BreakpointsForDimension1=t_e_6  Table=angular_velocity_pitch_6  InternalRulePriority=Speed  RndMeth=Simplest  InputSameDT=on
  1-D Lookup Table7 : Lookup_n-D  NumberOfTableDimensions=1  BreakpointsForDimension1=t_e_6  Table=angular_velocity_pitch_6  InternalRulePriority=Speed  RndMeth=Simplest  InputSameDT=on
  Add{,1..5} (6 alike) : Sum  Inputs=+-
  Clock : Clock
  Constant : Constant  Value=t_1_last
  Constant1 : Constant  Value=t_1_last+t_2_last
  Constant2 : Constant  Value=t_1_last+t_2_last+t_3_last
  Constant3 : Constant  Value=t_1_last+t_2_last+t_3_last+t_4_last
  Constant4 : Constant  Value=t_1_last+t_2_last+t_3_last+t_4_last+t_5_last
  Constant5 : Constant  Value=t_1_last+t_2_last+t_3_last+t_4_last+t_5_last+t_6_last
  Multiport Switch : MultiPortSwitch  Inputs=7
  Transfer Fcn : TransferFcn  Denominator=[1 1]
  pitch_d : Outport
  wires:
  1-D Lookup Table1/1 -> Multiport Switch/3
  1-D Lookup Table3/1 -> Multiport Switch/2
  Constant/1 -> Add/2
  Multiport Switch/1 -> Transfer Fcn/1
  SwitchSchedule/1 -> Multiport Switch/1
  Clock/1 -> Add5/1, Add4/1, Add3/1, Add2/1, Add1/1, Add/1, 1-D Lookup Table3/1
  Add/1 -> 1-D Lookup Table1/1
  1-D Lookup Table2/1 -> Multiport Switch/4
  Constant1/1 -> Add1/2
  Add1/1 -> 1-D Lookup Table2/1
  Constant2/1 -> Add2/2
  Add2/1 -> 1-D Lookup Table4/1
  1-D Lookup Table4/1 -> Multiport Switch/5
  Transfer Fcn/1 -> pitch_d/1
  Constant3/1 -> Add3/2
  Add3/1 -> 1-D Lookup Table5/1
  1-D Lookup Table5/1 -> Multiport Switch/6
  Add4/1 -> 1-D Lookup Table6/1
  Constant4/1 -> Add4/2
  1-D Lookup Table6/1 -> Multiport Switch/7
  Add5/1 -> 1-D Lookup Table7/1
  Constant5/1 -> Add5/2
  1-D Lookup Table7/1 -> Multiport Switch/8

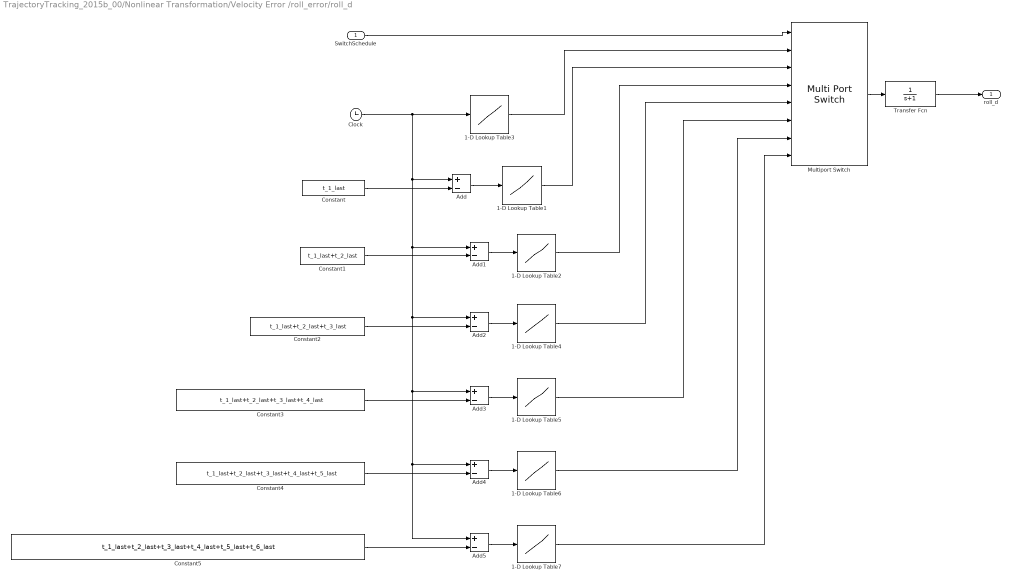
== system TrajectoryTracking_2015b_00/Nonlinear Transformation/Velocity Error /roll_error/roll_d ==
  SwitchSchedule : Inport
  1-D Lookup Table1 : Lookup_n-D  NumberOfTableDimensions=1  BreakpointsForDimension1=t_e_2  Table=angular_velocity_roll_2  InternalRulePriority=Speed  RndMeth=Simplest  InputSameDT=on
  1-D Lookup Table2 : Lookup_n-D  NumberOfTableDimensions=1  BreakpointsForDimension1=t_e_3  Table=angular_velocity_roll_3  InternalRulePriority=Speed  RndMeth=Simplest  InputSameDT=on
  1-D Lookup Table3 : Lookup_n-D  NumberOfTableDimensions=1  BreakpointsForDimension1=t_e_1  Table=angular_velocity_roll_1  InternalRulePriority=Speed  RndMeth=Simplest  InputSameDT=on
  1-D Lookup Table4 : Lookup_n-D  NumberOfTableDimensions=1  BreakpointsForDimension1=t_e_4  Table=angular_velocity_roll_4  InternalRulePriority=Speed  RndMeth=Simplest  InputSameDT=on
  1-D Lookup Table5 : Lookup_n-D  NumberOfTableDimensions=1  BreakpointsForDimension1=t_e_5  Table=angular_velocity_roll_5  InternalRulePriority=Speed  RndMeth=Simplest  InputSameDT=on
  1-D Lookup Table6 : Lookup_n-D  NumberOfTableDimensions=1  BreakpointsForDimension1=t_e_6  Table=angular_velocity_roll_6  InternalRulePriority=Speed  RndMeth=Simplest  InputSameDT=on
  1-D Lookup Table7 : Lookup_n-D  NumberOfTableDimensions=1  BreakpointsForDimension1=t_e_7  Table=angular_velocity_roll_7  InternalRulePriority=Speed  RndMeth=Simplest  InputSameDT=on
  Add{,1..5} (6 alike) : Sum  Inputs=+-
  Clock : Clock
  Constant : Constant  Value=t_1_last
  Constant1 : Constant  Value=t_1_last+t_2_last
  Constant2 : Constant  Value=t_1_last+t_2_last+t_3_last
  Constant3 : Constant  Value=t_1_last+t_2_last+t_3_last+t_4_last
  Constant4 : Constant  Value=t_1_last+t_2_last+t_3_last+t_4_last+t_5_last
  Constant5 : Constant  Value=t_1_last+t_2_last+t_3_last+t_4_last+t_5_last+t_6_last
  Multiport Switch : MultiPortSwitch  Inputs=7
  Transfer Fcn : TransferFcn  Denominator=[1 1]
  roll_d : Outport
  wires:
  1-D Lookup Table1/1 -> Multiport Switch/3
  1-D Lookup Table3/1 -> Multiport Switch/2
  Constant/1 -> Add/2
  Multiport Switch/1 -> Transfer Fcn/1
  SwitchSchedule/1 -> Multiport Switch/1
  Clock/1 -> Add5/1, Add4/1, Add3/1, Add2/1, Add1/1, Add/1, 1-D Lookup Table3/1
  Add/1 -> 1-D Lookup Table1/1
  Constant1/1 -> Add1/2
  Add1/1 -> 1-D Lookup Table2/1
  1-D Lookup Table2/1 -> Multiport Switch/4
  Add2/1 -> 1-D Lookup Table4/1
  Constant2/1 -> Add2/2
  1-D Lookup Table4/1 -> Multiport Switch/5
  Transfer Fcn/1 -> roll_d/1
  Constant3/1 -> Add3/2
  Add3/1 -> 1-D Lookup Table5/1
  1-D Lookup Table5/1 -> Multiport Switch/6
  Constant4/1 -> Add4/2
  Add4/1 -> 1-D Lookup Table6/1
  1-D Lookup Table6/1 -> Multiport Switch/7
  Add5/1 -> 1-D Lookup Table7/1
  Constant5/1 -> Add5/2
  1-D Lookup Table7/1 -> Multiport Switch/8

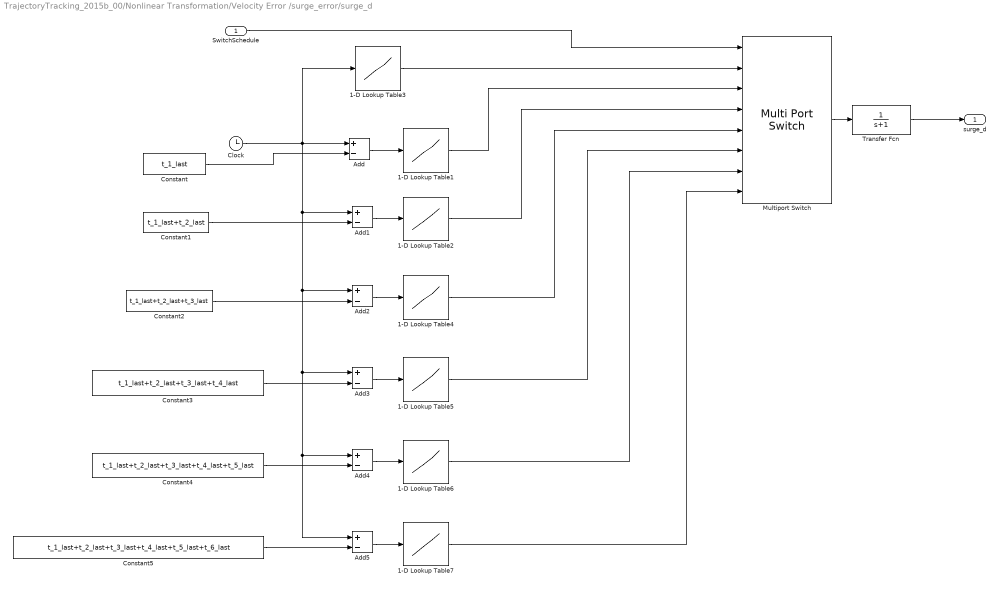
== system TrajectoryTracking_2015b_00/Nonlinear Transformation/Velocity Error /surge_error/surge_d ==
  SwitchSchedule : Inport
  1-D Lookup Table1 : Lookup_n-D  NumberOfTableDimensions=1  BreakpointsForDimension1=t_e_2  Table=linear_velocity_x_2  InternalRulePriority=Speed  RndMeth=Simplest  InputSameDT=on
  1-D Lookup Table2 : Lookup_n-D  NumberOfTableDimensions=1  BreakpointsForDimension1=t_e_3  Table=linear_velocity_x_3  InternalRulePriority=Speed  RndMeth=Simplest  InputSameDT=on
  1-D Lookup Table3 : Lookup_n-D  NumberOfTableDimensions=1  BreakpointsForDimension1=t_e_1  Table=linear_velocity_x_1  InternalRulePriority=Speed  RndMeth=Simplest  InputSameDT=on
  1-D Lookup Table4 : Lookup_n-D  NumberOfTableDimensions=1  BreakpointsForDimension1=t_e_4  Table=linear_velocity_x_4  InternalRulePriority=Speed  RndMeth=Simplest  InputSameDT=on
  1-D Lookup Table5 : Lookup_n-D  NumberOfTableDimensions=1  BreakpointsForDimension1=t_e_5  Table=linear_velocity_x_5  InternalRulePriority=Speed  RndMeth=Simplest  InputSameDT=on
  1-D Lookup Table6 : Lookup_n-D  NumberOfTableDimensions=1  BreakpointsForDimension1=t_e_6  Table=linear_velocity_x_6  InternalRulePriority=Speed  RndMeth=Simplest  InputSameDT=on
  1-D Lookup Table7 : Lookup_n-D  NumberOfTableDimensions=1  BreakpointsForDimension1=t_e_7  Table=linear_velocity_x_7  InternalRulePriority=Speed  RndMeth=Simplest  InputSameDT=on
  Add{,1..5} (6 alike) : Sum  Inputs=+-
  Clock : Clock
  Constant : Constant  Value=t_1_last
  Constant1 : Constant  Value=t_1_last+t_2_last
  Constant2 : Constant  Value=t_1_last+t_2_last+t_3_last
  Constant3 : Constant  Value=t_1_last+t_2_last+t_3_last+t_4_last
  Constant4 : Constant  Value=t_1_last+t_2_last+t_3_last+t_4_last+t_5_last
  Constant5 : Constant  Value=t_1_last+t_2_last+t_3_last+t_4_last+t_5_last+t_6_last
  Multiport Switch : MultiPortSwitch  Inputs=7
  Transfer Fcn : TransferFcn  Denominator=[1 1]
  surge_d : Outport
  wires:
  1-D Lookup Table1/1 -> Multiport Switch/3
  1-D Lookup Table3/1 -> Multiport Switch/2
  Constant/1 -> Add/2
  Multiport Switch/1 -> Transfer Fcn/1
  SwitchSchedule/1 -> Multiport Switch/1
  Clock/1 -> Add5/1, Add4/1, Add3/1, Add2/1, Add1/1, Add/1, 1-D Lookup Table3/1
  Add/1 -> 1-D Lookup Table1/1
  Constant1/1 -> Add1/2
  Add1/1 -> 1-D Lookup Table2/1
  1-D Lookup Table2/1 -> Multiport Switch/4
  Constant2/1 -> Add2/2
  Add2/1 -> 1-D Lookup Table4/1
  1-D Lookup Table4/1 -> Multiport Switch/5
  Transfer Fcn/1 -> surge_d/1
  Add3/1 -> 1-D Lookup Table5/1
  Constant3/1 -> Add3/2
  1-D Lookup Table5/1 -> Multiport Switch/6
  Constant4/1 -> Add4/2
  Add4/1 -> 1-D Lookup Table6/1
  1-D Lookup Table6/1 -> Multiport Switch/7
  Constant5/1 -> Add5/2
  Add5/1 -> 1-D Lookup Table7/1
  1-D Lookup Table7/1 -> Multiport Switch/8

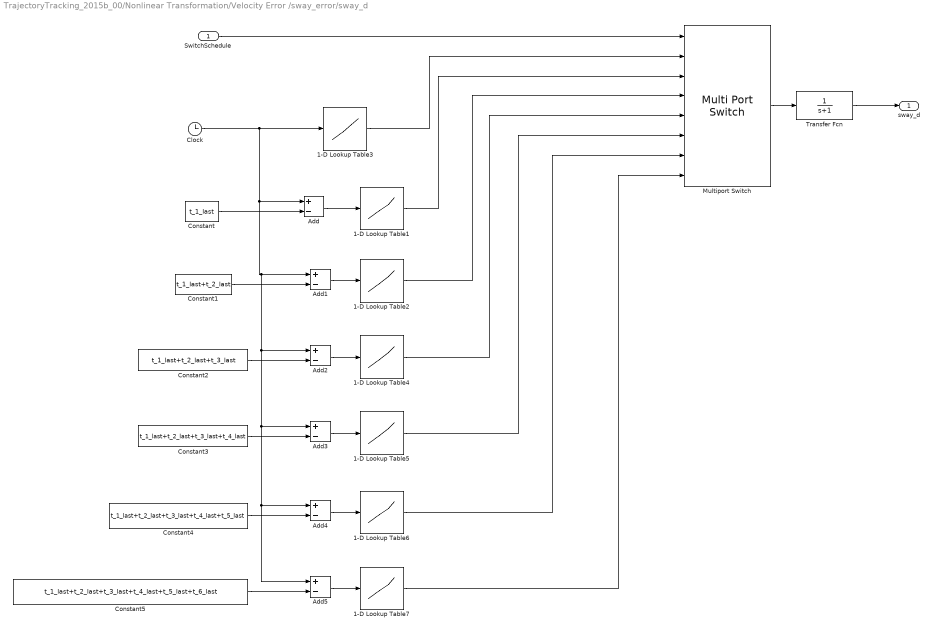
== system TrajectoryTracking_2015b_00/Nonlinear Transformation/Velocity Error /sway_error/sway_d ==
  SwitchSchedule : Inport
  1-D Lookup Table1 : Lookup_n-D  NumberOfTableDimensions=1  BreakpointsForDimension1=t_e_2  Table=linear_velocity_y_2  InternalRulePriority=Speed  RndMeth=Simplest  InputSameDT=on
  1-D Lookup Table2 : Lookup_n-D  NumberOfTableDimensions=1  BreakpointsForDimension1=t_e_3  Table=linear_velocity_y_3  InternalRulePriority=Speed  RndMeth=Simplest  InputSameDT=on
  1-D Lookup Table3 : Lookup_n-D  NumberOfTableDimensions=1  BreakpointsForDimension1=t_e_1  Table=linear_velocity_y_1  InternalRulePriority=Speed  RndMeth=Simplest  InputSameDT=on
  1-D Lookup Table4 : Lookup_n-D  NumberOfTableDimensions=1  BreakpointsForDimension1=t_e_4  Table=linear_velocity_y_4  InternalRulePriority=Speed  RndMeth=Simplest  InputSameDT=on
  1-D Lookup Table5 : Lookup_n-D  NumberOfTableDimensions=1  BreakpointsForDimension1=t_e_5  Table=linear_velocity_y_5  InternalRulePriority=Speed  RndMeth=Simplest  InputSameDT=on
  1-D Lookup Table6 : Lookup_n-D  NumberOfTableDimensions=1  BreakpointsForDimension1=t_e_6  Table=linear_velocity_y_6  InternalRulePriority=Speed  RndMeth=Simplest  InputSameDT=on
  1-D Lookup Table7 : Lookup_n-D  NumberOfTableDimensions=1  BreakpointsForDimension1=t_e_7  Table=linear_velocity_y_7  InternalRulePriority=Speed  RndMeth=Simplest  InputSameDT=on
  Add{,1..5} (6 alike) : Sum  Inputs=+-
  Clock : Clock
  Constant : Constant  Value=t_1_last
  Constant1 : Constant  Value=t_1_last+t_2_last
  Constant2 : Constant  Value=t_1_last+t_2_last+t_3_last
  Constant3 : Constant  Value=t_1_last+t_2_last+t_3_last+t_4_last
  Constant4 : Constant  Value=t_1_last+t_2_last+t_3_last+t_4_last+t_5_last
  Constant5 : Constant  Value=t_1_last+t_2_last+t_3_last+t_4_last+t_5_last+t_6_last
  Multiport Switch : MultiPortSwitch  Inputs=7
  Transfer Fcn : TransferFcn  Denominator=[1 1]
  sway_d : Outport
  wires:
  1-D Lookup Table1/1 -> Multiport Switch/3
  1-D Lookup Table3/1 -> Multiport Switch/2
  Constant/1 -> Add/2
  Multiport Switch/1 -> Transfer Fcn/1
  SwitchSchedule/1 -> Multiport Switch/1
  Clock/1 -> Add/1, Add5/1, Add4/1, Add3/1, Add2/1, Add1/1, 1-D Lookup Table3/1
  Add/1 -> 1-D Lookup Table1/1
  Constant1/1 -> Add1/2
  Add1/1 -> 1-D Lookup Table2/1
  1-D Lookup Table2/1 -> Multiport Switch/4
  Constant2/1 -> Add2/2
  Add2/1 -> 1-D Lookup Table4/1
  1-D Lookup Table4/1 -> Multiport Switch/5
  Transfer Fcn/1 -> sway_d/1
  Add3/1 -> 1-D Lookup Table5/1
  Constant3/1 -> Add3/2
  1-D Lookup Table5/1 -> Multiport Switch/6
  Constant4/1 -> Add4/2
  Add4/1 -> 1-D Lookup Table6/1
  1-D Lookup Table6/1 -> Multiport Switch/7
  Constant5/1 -> Add5/2
  Add5/1 -> 1-D Lookup Table7/1
  1-D Lookup Table7/1 -> Multiport Switch/8

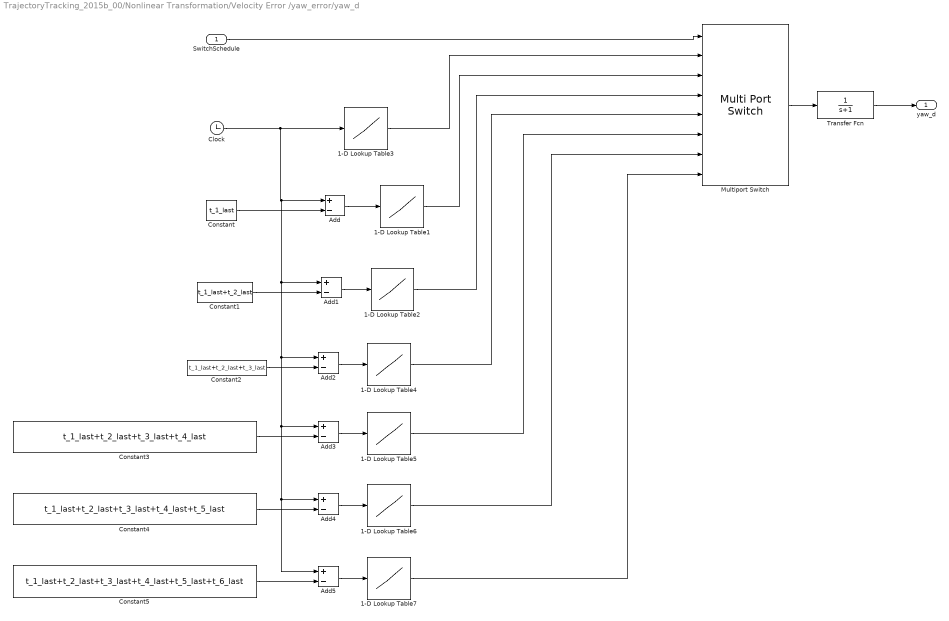
== system TrajectoryTracking_2015b_00/Nonlinear Transformation/Velocity Error /yaw_error/yaw_d ==
  SwitchSchedule : Inport
  1-D Lookup Table1 : Lookup_n-D  NumberOfTableDimensions=1  BreakpointsForDimension1=t_e_2  Table=angular_velocity_yaw_2  InternalRulePriority=Speed  RndMeth=Simplest  InputSameDT=on
  1-D Lookup Table2 : Lookup_n-D  NumberOfTableDimensions=1  BreakpointsForDimension1=t_e_3  Table=angular_velocity_yaw_3  InternalRulePriority=Speed  RndMeth=Simplest  InputSameDT=on
  1-D Lookup Table3 : Lookup_n-D  NumberOfTableDimensions=1  BreakpointsForDimension1=t_e_1  Table=angular_velocity_yaw_1  InternalRulePriority=Speed  RndMeth=Simplest  InputSameDT=on
  1-D Lookup Table4 : Lookup_n-D  NumberOfTableDimensions=1  BreakpointsForDimension1=t_e_4  Table=angular_velocity_yaw_4  InternalRulePriority=Speed  RndMeth=Simplest  InputSameDT=on
  1-D Lookup Table5 : Lookup_n-D  NumberOfTableDimensions=1  BreakpointsForDimension1=t_e_5  Table=angular_velocity_yaw_5  InternalRulePriority=Speed  RndMeth=Simplest  InputSameDT=on
  1-D Lookup Table6 : Lookup_n-D  NumberOfTableDimensions=1  BreakpointsForDimension1=t_e_6  Table=angular_velocity_yaw_6  InternalRulePriority=Speed  RndMeth=Simplest  InputSameDT=on
  1-D Lookup Table7 : Lookup_n-D  NumberOfTableDimensions=1  BreakpointsForDimension1=t_e_7  Table=angular_velocity_yaw_7  InternalRulePriority=Speed  RndMeth=Simplest  InputSameDT=on
  Add{,1..5} (6 alike) : Sum  Inputs=+-
  Clock : Clock
  Constant : Constant  Value=t_1_last
  Constant1 : Constant  Value=t_1_last+t_2_last
  Constant2 : Constant  Value=t_1_last+t_2_last+t_3_last
  Constant3 : Constant  Value=t_1_last+t_2_last+t_3_last+t_4_last
  Constant4 : Constant  Value=t_1_last+t_2_last+t_3_last+t_4_last+t_5_last
  Constant5 : Constant  Value=t_1_last+t_2_last+t_3_last+t_4_last+t_5_last+t_6_last
  Multiport Switch : MultiPortSwitch  Inputs=7
  Transfer Fcn : TransferFcn  Denominator=[1 1]
  yaw_d : Outport
  wires:
  1-D Lookup Table1/1 -> Multiport Switch/3
  1-D Lookup Table3/1 -> Multiport Switch/2
  Constant/1 -> Add/2
  Multiport Switch/1 -> Transfer Fcn/1
  SwitchSchedule/1 -> Multiport Switch/1
  Clock/1 -> Add5/1, Add4/1, Add3/1, Add2/1, Add1/1, Add/1, 1-D Lookup Table3/1
  Add/1 -> 1-D Lookup Table1/1
  1-D Lookup Table2/1 -> Multiport Switch/4
  Constant1/1 -> Add1/2
  Add1/1 -> 1-D Lookup Table2/1
  Constant2/1 -> Add2/2
  Add2/1 -> 1-D Lookup Table4/1
  Transfer Fcn/1 -> yaw_d/1
  Add3/1 -> 1-D Lookup Table5/1
  Constant3/1 -> Add3/2
  1-D Lookup Table4/1 -> Multiport Switch/5
  1-D Lookup Table5/1 -> Multiport Switch/6
  Add4/1 -> 1-D Lookup Table6/1
  Constant4/1 -> Add4/2
  1-D Lookup Table6/1 -> Multiport Switch/7
  Constant5/1 -> Add5/2
  Add5/1 -> 1-D Lookup Table7/1
  1-D Lookup Table7/1 -> Multiport Switch/8

== system TrajectoryTracking_2015b_00/Underwater Robot System/Underwater Robot System/Dynamic2Kinematic(angular velocity)/Initial Integration Phi ==
  Constant : Constant  Value=0
  Initial Phi Integration Value : Outport
  wires:
  Constant/1 -> Initial Phi Integration Value/1

== system TrajectoryTracking_2015b_00/Underwater Robot System/Underwater Robot System/Dynamic2Kinematic(angular velocity)/Initial Integration Value Generation Psi ==
  Constant : Constant  Value=0
  Initial Orientation Integration Value : Outport
  wires:
  Constant/1 -> Initial Orientation Integration Value/1
